simulink model "UBoot_LowLevelRegler"  (R2014a)
settings: Solver=ode45  StartTime=0.0  StopTime=inf  RelTol=1e-3
libraries: simulink x2
settings Model: Creator=Jonis  LastModifiedBy=Jonis
settings DebuggingCC: UnderspecifiedInitializationDetection=Classic

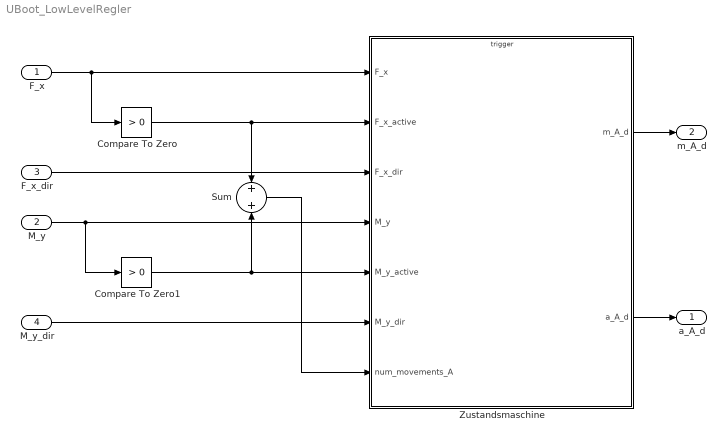
== system UBoot_LowLevelRegler ==
  F_x : Inport
  M_y : Inport  Port=2
  F_x_dir : Inport  Port=3
  M_y_dir : Inport  Port=4
  Compare To Zero : simulink/Logic and Bit Operations/Compare To Zero  relop=>  OutDataTypeStr=boolean
  Compare To Zero1 : simulink/Logic and Bit Operations/Compare To Zero  relop=>  OutDataTypeStr=boolean
  Sum : Sum
  Zustandsmaschine : Stateflow chart  TreatAsAtomicUnit=on
  a_A_d : Outport
  m_A_d : Outport  Port=2
  wires:
  F_x/1 -> Zustandsmaschine/1(F_x), Compare To Zero/1
  Compare To Zero/1 -> Zustandsmaschine/2(F_x_active), Sum/1
  M_y/1 -> Zustandsmaschine/4(M_y), Compare To Zero1/1
  Compare To Zero1/1 -> Sum/2, Zustandsmaschine/5(M_y_active)
  Zustandsmaschine/1(m_A_d) -> m_A_d/1
  Zustandsmaschine/2(a_A_d) -> a_A_d/1
  Sum/1 -> Zustandsmaschine/7(num_movements_A)
  F_x_dir/1 -> Zustandsmaschine/3(F_x_dir)
  M_y_dir/1 -> Zustandsmaschine/6(M_y_dir)

== stateflow chart UBoot_LowLevelRegler/Zustandsmaschine ==
  state two_directions
    state postive_force_positive_torque
      state two_pp_positive_force
        entry: a_A_d = A_angle_positive_force;
        m_A_d = F_x;
      state two_pp_positive_torque
        entry: a_A_d = A_angle_positive_torque;
        m_A_d = M_y;
      two_pp_positive_torque -> two_pp_positive_force : after(deadband(A_angle_positive_force-A_angle_positive_torque) + (M_y/(F_x + M_y))*switch_time, s)
      (default) -> two_pp_positive_force
      two_pp_positive_force -> two_pp_positive_torque : after(deadband(A_angle_positive_force-A_angle_positive_torque) + (F_x/(F_x + M_y))*switch_time, s)
    state postive_force_negative_torque
    state negative_force_positive_torque
    state negative_force_negative_torque
    postive_force_positive_torque -> (junction 45) : [F_x_dir == 0 || M_y_dir == 0]
    (junction 30) -> postive_force_positive_torque [order 1] : [M_y_dir == 1]
    (junction 30) -> postive_force_negative_torque [order 2] : [M_y_dir == 0]
    postive_force_negative_torque -> (junction 45) : [F_x_dir == 0 || M_y_dir == 1]
    (junction 29) -> (junction 30) [order 2] : [F_x_dir == 1]
    negative_force_positive_torque -> (junction 45) : [F_x_dir == 1 || M_y_dir == 0]
    (junction 45) -> (junction 29) : after(switch_time, s)
    negative_force_negative_torque -> (junction 45) : [F_x_dir == 1 || M_y_dir == 1]
    (default) -> (junction 29)
    (junction 29) -> (junction 31) [order 1] : [F_x_dir == 0]
    (junction 31) -> negative_force_positive_torque [order 1] : [M_y_dir == 1]
    (junction 31) -> negative_force_negative_torque [order 2] : [M_y_dir == 0]
  state one_direction
    state positive_force
      entry: a_A_d = A_angle_positive_force;
      m_A_d = F_x;
    state negative_force
      entry: a_A_d = A_angle_negative_force;
      m_A_d = F_x;
    state positive_torque
      entry: a_A_d = A_angle_positive_torque;
      m_A_d = M_y;
    state negative_torque
      entry: a_A_d = A_angle_negative_torque;
      m_A_d = M_y;
    (junction 23) -> (junction 13) : after(switch_time,s)
    (default) -> (junction 13)
    (junction 13) -> positive_force [order 1] : [F_x_active && F_x_dir == 1]
    positive_force -> (junction 23)
    negative_force -> (junction 23)
    (junction 13) -> negative_force [order 2] : [F_x_active && F_x_dir == 0]
    positive_torque -> (junction 23)
    (junction 13) -> negative_torque [order 4] : [M_y_active && M_y_dir == 0]
    (junction 13) -> positive_torque [order 3] : [M_y_active && M_y_dir == 1]
    negative_torque -> (junction 23)
  state no_movement
    entry: a_A_d = 0;
    m_A_d = 0;
  (default) -> no_movement
  one_direction -> two_directions [order 2] : [num_movements_A > 1]
  no_movement -> one_direction : [num_movements_A > 0]
  one_direction -> no_movement [order 1] : [num_movements_A < 1]
  two_directions -> one_direction : [num_movements_A < 2]
  data: angle function_input double; dead_time function_output double; A_angle_negative_force constant double; A_angle_negative_torque constant double; A_angle_positive_force constant double; A_angle_positive_torque constant double; F_x input; F_x_active input; F_x_dir input; M_y input; M_y_active input; M_y_dir input; num_movements_A input; switch_time constant double; m_A_d output double; a_A_d output double
  events: s input RISING_EDGE_EVENT
  function dead_time   = deadband( angle ):
    | function dead_time   = deadband( angle )
    | %UNTITLED Summary of this function goes here
    | %   Detailed explanation goes here
    |     dead_time = 0.0005 + angle/200 * 0.01;
    | 
    | end
